simulink model "Punto_6c"  (R2020a)
settings: Solver=VariableStepAuto  StartTime=0.0  StopTime=20.0  RelTol=1e-3
undefined symbols (not defined in the file): A, B
libraries: simulink x2
settings Model: Creator=nicoquintero  LastModifiedBy=nicoquintero

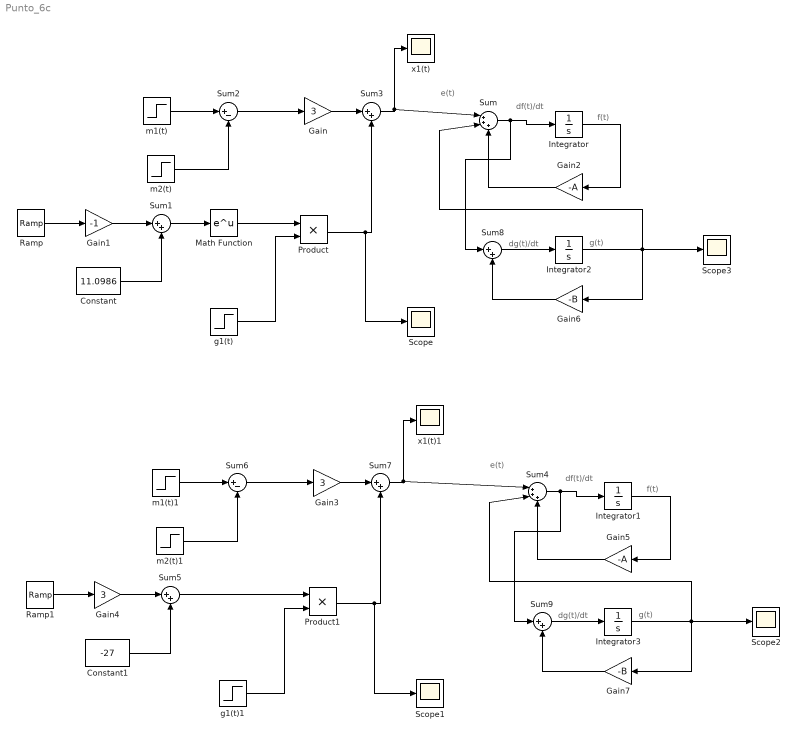
== system Punto_6c ==
  note: df(t)/dt
  note: g(t)
  note: f(t)
  note: dg(t)/dt
  note: e(t)
  note: dg(t)/dt
  note: f(t)
  note: df(t)/dt
  note: g(t)
  note: e(t)
  Constant : Constant  Value=11.0986
  Constant1 : Constant  Value=-27
  Gain : Gain  Gain=3
  Gain1 : Gain  Gain=-1
  Gain2 : Gain  Gain=-A
  Gain3 : Gain  Gain=3
  Gain4 : Gain  Gain=3
  Gain5 : Gain  Gain=-A
  Gain6 : Gain  Gain=-B
  Gain7 : Gain  Gain=-B
  Integrator{,1..3} (4 alike) : Integrator
  Math Function : Math  SaturateOnIntegerOverflow=on
  Product : Product
  Product1 : Product
  Ramp : simulink/Sources/Ramp  slope=1  start=0  InitialOutput=0
  Ramp1 : simulink/Sources/Ramp  slope=1  start=0  InitialOutput=0
  Scope{,1..3} (4 alike) : Scope
  Sum : Sum  Inputs=|+++
  Sum{1,3,5,7..9} (6 alike) : Sum  Inputs=|++
  Sum2 : Sum  Inputs=|+-
  Sum4 : Sum  Inputs=|+++
  Sum6 : Sum  Inputs=|+-
  g1(t) : Step  Time=10  SampleTime=0
  g1(t)1 : Step  Time=10  SampleTime=0
  m1(t) : Step  Time=0  SampleTime=0
  m1(t)1 : Step  Time=0  SampleTime=0
  m2(t) : Step  Time=10  SampleTime=0
  m2(t)1 : Step  Time=10  SampleTime=0
  x1(t) : Scope
  x1(t)1 : Scope
  wires:
  Sum1/1 -> Math Function/1
  Constant1/1 -> Sum5/2
  g1(t)/1 -> Product/2
  Gain3/1 -> Sum7/1
  m2(t)/1 -> Sum2/2
  Constant/1 -> Sum1/2
  Sum6/1 -> Gain3/1
  Gain1/1 -> Sum1/1
  Ramp/1 -> Gain1/1
  m1(t)/1 -> Sum2/1
  Ramp1/1 -> Gain4/1
  Gain/1 -> Sum3/1
  m1(t)1/1 -> Sum6/1
  Sum5/1 -> Product1/1
  Product1/1 -> Scope1/1, Sum7/2
  m2(t)1/1 -> Sum6/2
  Math Function/1 -> Product/1
  Product/1 -> Scope/1, Sum3/2
  Gain4/1 -> Sum5/1
  Sum2/1 -> Gain/1
  g1(t)1/1 -> Product1/2
  Gain2/1 -> Sum/3
  Sum/1 -> Sum8/1, Integrator/1
  Gain6/1 -> Sum8/2
  Sum8/1 -> Integrator2/1
  Integrator2/1 -> Sum/2, Scope3/1, Gain6/1
  Integrator/1 -> Gain2/1
  Sum3/1 -> Sum/1, x1(t)/1
  Integrator3/1 -> Sum4/2, Scope2/1, Gain7/1
  Integrator1/1 -> Gain5/1
  Gain5/1 -> Sum4/3
  Sum4/1 -> Sum9/1, Integrator1/1
  Gain7/1 -> Sum9/2
  Sum9/1 -> Integrator3/1
  Sum7/1 -> Sum4/1, x1(t)1/1
